simulink model "BLDC"  (R2021a)
settings: Solver=VariableStepAuto  StartTime=0.0  StopTime=1  RelTol=1e-3
settings Model: Creator=serkan  LastModifiedBy=serkan

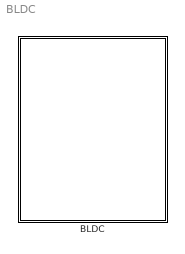
== system BLDC ==
  BLDC : Subsystem  mask{R=1.45, L=1e-3}
      mask prompts: R "Direnc"; L "Enduktans"

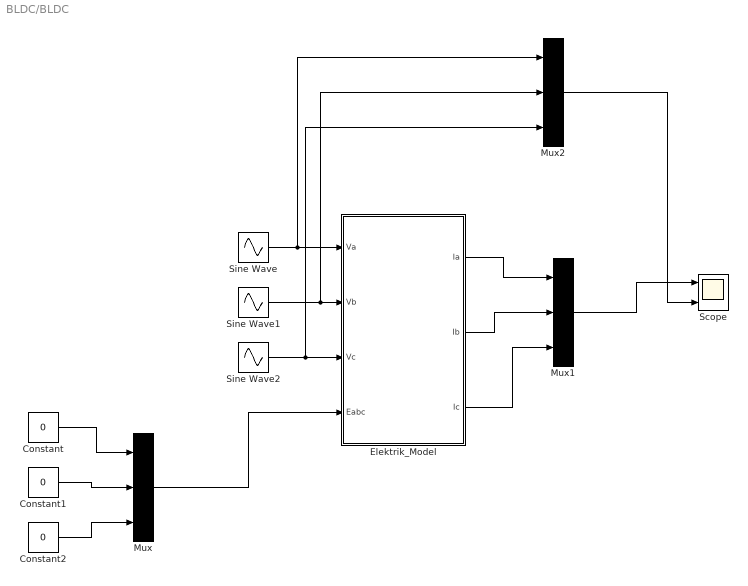
== system BLDC/BLDC ==
  Constant : Constant  Value=0
  Constant1 : Constant  Value=0
  Constant2 : Constant  Value=0
  Elektrik_Model : Subsystem
  Mux : Mux  Inputs=3
  Mux1 : Mux  Inputs=3
  Mux2 : Mux  Inputs=3
  Scope : Scope  NumInputPorts=2
  Sine Wave : Sin  Amplitude=5  Frequency=2*pi*50  SampleTime=1e-5
  Sine Wave1 : Sin  Amplitude=5  Frequency=2*pi*50  Phase=-2*pi/3  SampleTime=1e-5
  Sine Wave2 : Sin  Amplitude=5  Frequency=2*pi*50  Phase=2*pi/3  SampleTime=1e-5
  wires:
  Sine Wave/1 -> Mux2/1, Elektrik_Model/1(Va)
  Sine Wave1/1 -> Mux2/2, Elektrik_Model/2(Vb)
  Sine Wave2/1 -> Mux2/3, Elektrik_Model/3(Vc)
  Constant/1 -> Mux/1
  Constant1/1 -> Mux/2
  Constant2/1 -> Mux/3
  Mux/1 -> Elektrik_Model/4(Eabc)
  Elektrik_Model/1(Ia) -> Mux1/1
  Elektrik_Model/2(Ib) -> Mux1/2
  Elektrik_Model/3(Ic) -> Mux1/3
  Mux1/1 -> Scope/1
  Mux2/1 -> Scope/2

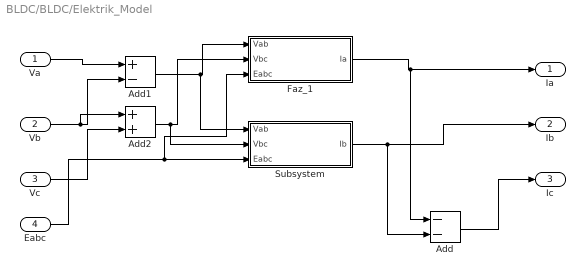
== system BLDC/BLDC/Elektrik_Model ==
  Va : Inport
  Vb : Inport  Port=2
  Vc : Inport  Port=3
  Eabc : Inport  Port=4
  Add : Sum  Inputs=--
  Add1 : Sum  Inputs=+-
  Add2 : Sum
  Faz_1 : Subsystem
  Subsystem : Subsystem
  Ia : Outport
  Ib : Outport  Port=2
  Ic : Outport  Port=3
  wires:
  Faz_1/1(Ia) -> Add/1, Ia/1
  Subsystem/1(Ib) -> Add/2, Ib/1
  Add/1 -> Ic/1
  Va/1 -> Add1/1
  Vb/1 -> Add2/1, Add1/2
  Add1/1 -> Subsystem/1(Vab), Faz_1/1(Vab)
  Vc/1 -> Add2/2
  Add2/1 -> Subsystem/2(Vbc), Faz_1/2(Vbc)
  Eabc/1 -> Faz_1/3(Eabc), Subsystem/3(Eabc)

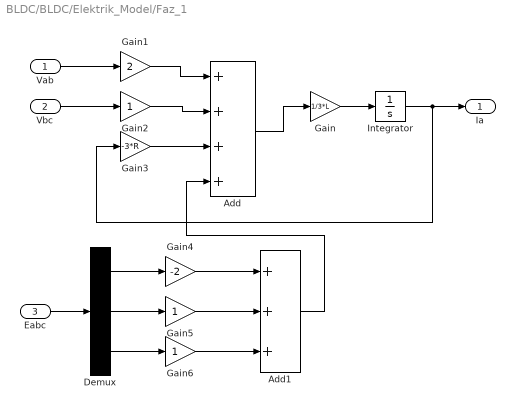
== system BLDC/BLDC/Elektrik_Model/Faz_1 ==
  Vab : Inport
  Vbc : Inport  Port=2
  Eabc : Inport  Port=3
  Add : Sum  Inputs=++++
  Add1 : Sum  Inputs=+++
  Demux : Demux  Outputs=3
  Gain : Gain  Gain=1/3*L
  Gain1 : Gain  Gain=2
  Gain2 : Gain
  Gain3 : Gain  Gain=-3*R
  Gain4 : Gain  Gain=-2
  Gain5 : Gain
  Gain6 : Gain
  Integrator : Integrator
  Ia : Outport
  wires:
  Gain/1 -> Integrator/1
  Integrator/1 -> Gain3/1, Ia/1
  Vbc/1 -> Gain2/1
  Vab/1 -> Gain1/1
  Gain1/1 -> Add/1
  Gain2/1 -> Add/2
  Gain3/1 -> Add/3
  Eabc/1 -> Demux/1
  Demux/1 -> Gain4/1
  Demux/2 -> Gain5/1
  Demux/3 -> Gain6/1
  Gain4/1 -> Add1/1
  Gain5/1 -> Add1/2
  Gain6/1 -> Add1/3
  Add/1 -> Gain/1
  Add1/1 -> Add/4

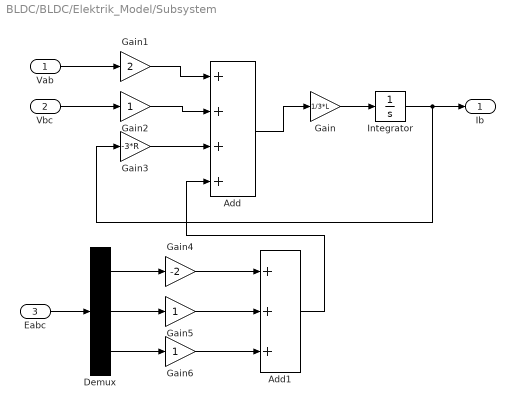
== system BLDC/BLDC/Elektrik_Model/Subsystem ==
  Vab : Inport
  Vbc : Inport  Port=2
  Eabc : Inport  Port=3
  Add : Sum  Inputs=++++
  Add1 : Sum  Inputs=+++
  Demux : Demux  Outputs=3
  Gain : Gain  Gain=1/3*L
  Gain1 : Gain  Gain=2
  Gain2 : Gain
  Gain3 : Gain  Gain=-3*R
  Gain4 : Gain  Gain=-2
  Gain5 : Gain
  Gain6 : Gain
  Integrator : Integrator
  Ib : Outport
  wires:
  Eabc/1 -> Demux/1
  Vbc/1 -> Gain2/1
  Gain3/1 -> Add/3
  Demux/1 -> Gain4/1
  Add1/1 -> Add/4
  Vab/1 -> Gain1/1
  Add/1 -> Gain/1
  Gain/1 -> Integrator/1
  Demux/3 -> Gain6/1
  Gain5/1 -> Add1/2
  Demux/2 -> Gain5/1
  Gain2/1 -> Add/2
  Integrator/1 -> Gain3/1, Ib/1
  Gain4/1 -> Add1/1
  Gain6/1 -> Add1/3
  Gain1/1 -> Add/1
